simulink model "untitled"  (R2019b)
settings: Solver=VariableStepAuto  StartTime=0.0  StopTime=50  RelTol=1e-3
settings Model: Creator=zoyil  LastModifiedBy=forest
settings DataIOCC: ReturnWorkspaceOutputs=off
settings DebuggingCC: ArithmeticOperatorsInVariantConditions=warning
settings SFSimCC: SimUseLocalCustomCode=off  CustomCodeUndefinedFunction=UseInterfaceOnly
settings RTWCC: RTWUseLocalCustomCode=off
settings CodeAppCC: StateflowObjectComments=on

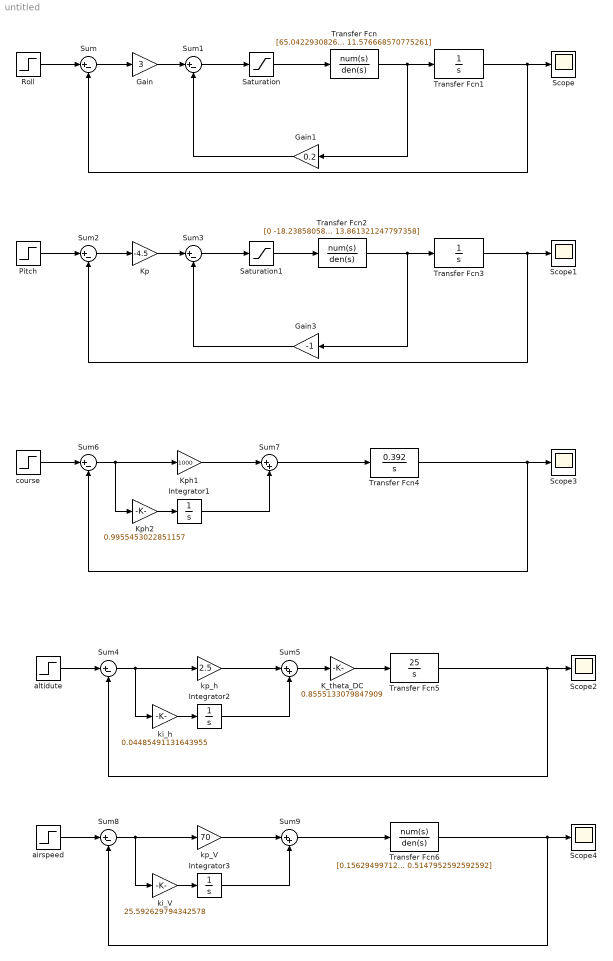
== system untitled ==
  Gain : Gain  Gain=3
  Gain1 : Gain  Gain=0.2
  Gain3 : Gain  Gain=-1
  Integrator1 : Integrator
  Integrator2 : Integrator
  Integrator3 : Integrator
  K_theta_DC : Gain  Gain=0.8555133079847909
  Kp : Gain  Gain=-4.5
  Kph1 : Gain  Gain=1000
  Kph2 : Gain  Gain=0.9955453022851157
  Pitch : Step  Time=0  SampleTime=0
  Roll : Step  Time=0  SampleTime=0
  Saturation : Saturate  UpperLimit=45  LowerLimit=-45
  Saturation1 : Saturate  UpperLimit=45  LowerLimit=-45
  Scope{,1..4} (5 alike) : Scope
  Sum{,1..4,6,8} (7 alike) : Sum  Inputs=|+-
  Sum5 : Sum  Inputs=|++
  Sum7 : Sum  Inputs=|++
  Sum9 : Sum  Inputs=|++
  Transfer Fcn : TransferFcn  Numerator=[65.04229308262757]  Denominator=[1 11.576668570775261]
  Transfer Fcn1 : TransferFcn  Denominator=[0 1 0]
  Transfer Fcn2 : TransferFcn  Numerator=[0 -18.23858058920705 0]  Denominator=[1 0.4988499835844141 13.861321247797358]
  Transfer Fcn3 : TransferFcn  Denominator=[0 1 0]
  Transfer Fcn4 : TransferFcn  Numerator=[0.392]  Denominator=[0 1 0]
  Transfer Fcn5 : TransferFcn  Numerator=[25]  Denominator=[0 1 0]
  Transfer Fcn6 : TransferFcn  Numerator=[0.15629499712000003]  Denominator=[0 1 0.5147952592592592]
  airspeed : Step  Time=0  SampleTime=0
  altidute : Step  Time=0  SampleTime=0
  course : Step  Time=0  SampleTime=0
  ki_V : Gain  Gain=25.592629794342578
  ki_h : Gain  Gain=0.04485491131643955
  kp_V : Gain  Gain=70
  kp_h : Gain  Gain=2.5
  wires:
  Sum/1 -> Gain/1
  Gain/1 -> Sum1/1
  Sum1/1 -> Saturation/1
  Saturation/1 -> Transfer Fcn/1
  Transfer Fcn/1 -> Gain1/1, Transfer Fcn1/1
  Gain1/1 -> Sum1/2
  Roll/1 -> Sum/1
  Transfer Fcn1/1 -> Scope/1, Sum/2
  Sum2/1 -> Kp/1
  Kp/1 -> Sum3/1
  Sum3/1 -> Saturation1/1
  Saturation1/1 -> Transfer Fcn2/1
  Transfer Fcn2/1 -> Gain3/1, Transfer Fcn3/1
  Gain3/1 -> Sum3/2
  Pitch/1 -> Sum2/1
  Transfer Fcn3/1 -> Scope1/1, Sum2/2
  Sum6/1 -> Kph2/1, Kph1/1
  Kph1/1 -> Sum7/1
  Sum7/1 -> Transfer Fcn4/1
  course/1 -> Sum6/1
  Transfer Fcn4/1 -> Scope3/1, Sum6/2
  Integrator1/1 -> Sum7/2
  Kph2/1 -> Integrator1/1
  Sum4/1 -> ki_h/1, kp_h/1
  kp_h/1 -> Sum5/1
  Sum5/1 -> K_theta_DC/1
  altidute/1 -> Sum4/1
  Transfer Fcn5/1 -> Scope2/1, Sum4/2
  Integrator2/1 -> Sum5/2
  ki_h/1 -> Integrator2/1
  K_theta_DC/1 -> Transfer Fcn5/1
  Integrator3/1 -> Sum9/2
  ki_V/1 -> Integrator3/1
  Transfer Fcn6/1 -> Scope4/1, Sum8/2
  airspeed/1 -> Sum8/1
  Sum8/1 -> ki_V/1, kp_V/1
  kp_V/1 -> Sum9/1
  Sum9/1 -> Transfer Fcn6/1
